simulink model "main_savepoint"  (R2021a)
settings: Solver=VariableStepAuto  StartTime=0.0  StopTime=60  RelTol=1e-3
undefined symbols (not defined in the file or in its folder): Earth, WGS84
libraries: pid_lib x6, dspvision x5, dspindex x2, aerolibfltsims x1, aerolibtransform2 x1, dspsnks4 x1, simulink x1
settings Model: Creator=ZumoArthicha  LastModifiedBy=ZumoArthicha

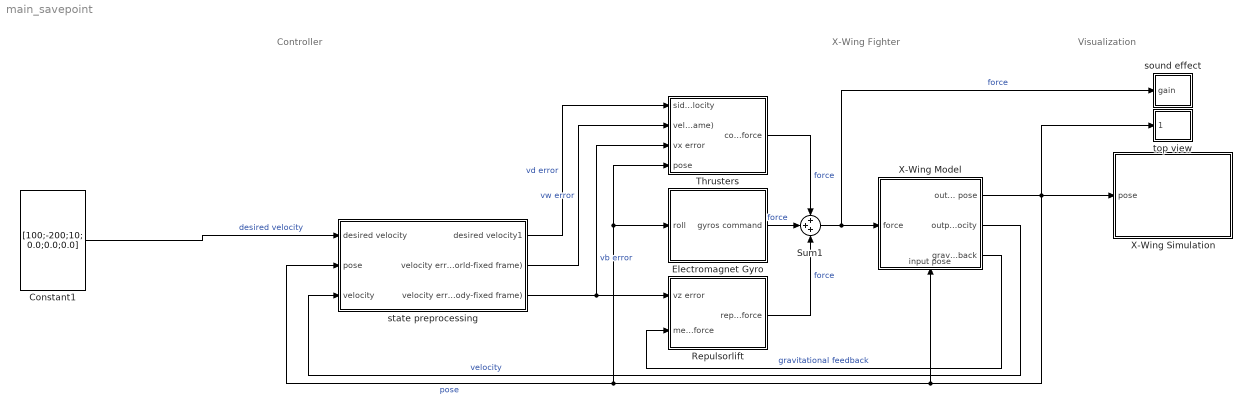
== system main_savepoint ==
  note: Controller
  note: Visualization
  note: X-Wing Fighter
  Constant1 : Constant  Value=[100;-200;10; 0.0;0.0;0.0]  VectorParams1D=off
  Electromagnet Gyro : Subsystem
      mask Display: image(imread("pictures/electromagneticgyro.PNG"))
  Repulsorlift : Subsystem
      mask Display: image(imread("pictures/repulserlift.PNG"))
  Sum1 : Sum  Inputs=+++
  Thrusters : Subsystem
      mask Display: image(imread("pictures/thrusters.PNG"))
  X-Wing Model : Subsystem
      settings: PortSchema="{\"entries\":[{\"content\":{\"sides\":[{\"content\":{\"connectorIds\":[\"In1\"]},\"type\":\"ConnectorPlacement.EquallySpacedRectSide\",\"uuid\":\"9b8fdf7d-c3f6-4599-b802-210579db8a0c\"},{\"content\":{\"connectorIds\":[\"Out1\",\"Out2\",\"Out3\"],\"side\":\"RIGHT\"},\"type\":\"ConnectorPlacement.EquallySpacedRectSide\",\"uuid\":\"64fce1f1-7921-46e2-bebf-614926f0f3ad\"},{\"content\":{\"connectorIds\":[],\"side\":\"TOP\"},\"type\":\"ConnectorPlacement.EquallySpacedRectSide\",\"uuid\":\"e545f28f-71e6-4ea6-95f8-1eb7e380d19b\"},{\"content\":{\"connectorIds\":[\"In2\"],\"side\":\"BOTTOM\"},\"type\":\"ConnectorPlacement.EquallySpacedRectSide\",\"uuid\":\"bfd9a8ec-cd4d-4e0d-ab0a-253386349908\"}]},\"type\":\"ConnectorPlacement.EquallySpacedConnector\",\"uuid\":\"b40ebf44-1443-4f81-b67e-9daee8e56b53\"}],\"packageUris\":[\"http://schema.mathworks.com/mf0/Connector/R2020b\"],\"version\":\"1.0\"}"
      mask Display: image(imread("pictures/simplified_model.png"))
  X-Wing Simulation : Subsystem
      mask Display: image(imread("pictures/simulation.PNG"))
  sound effect : Subsystem
      mask Display: image(imread("pictures/audio.PNG"))
  state preprocessing : Subsystem
  top view : Subsystem
      mask Display: image(imread("pictures/xy_graph.png"))
  wires:
  X-Wing Model/1(output pose) -> state preprocessing/2(pose), Electromagnet Gyro/1(roll), Thrusters/4(pose), X-Wing Model/2(input pose), X-Wing Simulation/1(pose), top view/1(" ")  "pose"
  X-Wing Model/3(gravitational force feedback) -> Repulsorlift/2(measured gravity force)  "gravitational feedback"
  Thrusters/1(combined thrusters force) -> Sum1/1  "force"
  Sum1/1 -> sound effect/1(gain), X-Wing Model/1(force)  "force"
  Electromagnet Gyro/1(gyros command) -> Sum1/2  "force"
  Repulsorlift/1(repulsorlift force) -> Sum1/3  "force"
  state preprocessing/3(velocity error (body-fixed frame)) -> Thrusters/3(vx error), Repulsorlift/1(vz error)  "vb error"
  X-Wing Model/2(output veloocity) -> state preprocessing/3(velocity)  "velocity"
  Constant1/1 -> state preprocessing/1(desired velocity)  "desired velocity"
  state preprocessing/1(desired velocity1) -> Thrusters/1(sideway velocity)  "vd error"
  state preprocessing/2(velocity error (world-fixed frame)) -> Thrusters/2(velocity error (world-fixed frame))  "vw error"

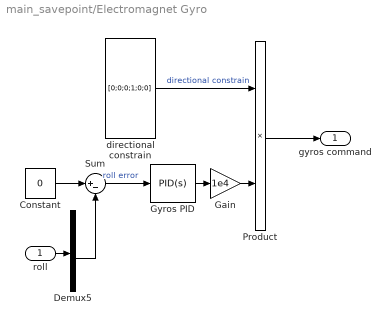
== system main_savepoint/Electromagnet Gyro ==
  roll : Inport
  Constant : Constant  Value=0
  Demux5 : Demux  Outputs=6
  Gain : Gain  Gain=1e4
  Gyros PID : pid_lib/PID Controller  Controller=PID  Form=Parallel  TimeDomain=Continuous-time  UseExternalTs=off  SampleTime=-1  IntegratorMethod=Forward Euler  FilterMethod=Forward Euler  ControllerParametersSource=internal  P=0.1  I=0  D=1  UseFilter=on  N=100  TunerSelectOption=Transfer Function Based (PID Tuner App)  InitialConditionSource=internal  InitialConditionForIntegrator=0  InitialConditionForFilter=0  DifferentiatorICPrevScaledInput=0  ExternalReset=none  TrackingMode=off  Kt=1  LimitOutput=off  SatLimitsSource=internal  UpperSaturationLimit=inf  LowerSaturationLimit=-inf  LinearizeAsGain=on  AntiWindupMode=none  Kb=1  POutMin=[]  POutMax=[]  IOutMin=[]  IOutMax=[]  DOutMin=[]  DOutMax=[]  NOutMin=[]  NOutMax=[]  SumOutMin=[]  SumOutMax=[]  SaturationOutMin=[]  SaturationOutMax=[]  PParamMin=[]  PParamMax=[]  IParamMin=[]  IParamMax=[]  DParamMin=[]  DParamMax=[]  NParamMin=[]  NParamMax=[]  KbParamMin=[]  KbParamMax=[]  KtParamMin=[]  KtParamMax=[]  KbOutMin=[]  KbOutMax=[]  KtOutMin=[]  KtOutMax=[]  IntegratorOutMin=[]  IntegratorOutMax=[]  FilterOutMin=[]  FilterOutMax=[]  SumI1OutMin=[]  SumI1OutMax=[]  SumI2OutMin=[]  SumI2OutMax=[]  SumI3OutMin=[]  SumI3OutMax=[]  SumI4OutMin=[]  SumI4OutMax=[]  SumDOutMin=[]  SumDOutMax=[]  DifferentiatorOutMin=[]  DifferentiatorOutMax=[]  FilterDiffOutCoefMin=[]  FilterDiffOutCoefMax=[]  ReciprocalOutMin=[]  ReciprocalOutMax=[]  SumDenOutMin=[]  SumDenOutMax=[]  SumNumOutMin=[]  SumNumOutMax=[]  DivideOutMin=[]  DivideOutMax=[]  UdiffTsProdOutMin=[]  UdiffTsProdOutMax=[]  NTsProdOutMin=[]  NTsProdOutMax=[]  UintegralTsProdOutMin=[]  UintegralTsProdOutMax=[]  UngainTsProdOutMin=[]  UngainTsProdOutMax=[]  IntegratorContinuousStateAttributes=''  IntegratorStateMustResolveToSignalObject=off  IntegratorRTWStateStorageClass=Auto  FilterContinuousStateAttributes=''  FilterStateMustResolveToSignalObject=off  FilterRTWStateStorageClass=Auto  ParallelPVariant=InternalParameters  IdealPVariant=Disabled  IVariant=InternalParameters  DVariant=InternalParameters  IntegratorVariant=Continuous  SatVariant=Disabled  AWVariant=Passthrough  PCopyVariant=Disabled  TRVariant=Disabled  FdbkBlocksVariant=Forward  IdealPFdbkVariant=Disabled  SatFdbkVariant=Disabled  DerivativeFilterVariant=ContFilter  NVariant=InternalParameters  NCopyVariant=Disabled  FilterICVariant=InternalICsFilter  IntegratorICVariant=InternalICs  ExternalResetVariant=Disabled  TRSumVariant=Passthrough  SumFdbkVariant=Disabled  SumVariant=Sum_PID  TsampFilterVariant=InternalTs  TsampNgainVariant=Passthrough  TsampIntegralVariant=Passthrough  ExternalSaturationOutDataTypeStr=Inherit: Same as second input
  Product : Product
  Sum : Sum  Inputs=|+-
  directional constrain : Constant  Value=[0;0;0;1;0;0]  VectorParams1D=off
  gyros command : Outport  PortDimensions=6
  wires:
  directional constrain/1 -> Product/1  "directional constrain"
  Gyros PID/1 -> Gain/1
  Product/1 -> gyros command/1
  Gain/1 -> Product/2
  Sum/1 -> Gyros PID/1  "roll error"
  Constant/1 -> Sum/1
  roll/1 -> Demux5/1
  Demux5/4 -> Sum/2

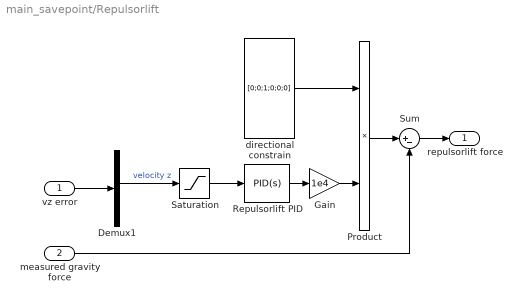
== system main_savepoint/Repulsorlift ==
  vz error : Inport
  measured gravity force : Inport  Port=2
  Demux1 : Demux  Outputs=6
  Gain : Gain  Gain=1e4
  Product : Product
  Repulsorlift PID : pid_lib/PID Controller  Controller=PID  Form=Parallel  TimeDomain=Continuous-time  UseExternalTs=off  SampleTime=-1  IntegratorMethod=Forward Euler  FilterMethod=Forward Euler  ControllerParametersSource=internal  P=0.05  I=0  D=1  UseFilter=on  N=100  TunerSelectOption=Transfer Function Based (PID Tuner App)  InitialConditionSource=internal  InitialConditionForIntegrator=0  InitialConditionForFilter=0  DifferentiatorICPrevScaledInput=0  ExternalReset=none  TrackingMode=off  Kt=1  LimitOutput=off  SatLimitsSource=internal  UpperSaturationLimit=inf  LowerSaturationLimit=-inf  LinearizeAsGain=on  AntiWindupMode=none  Kb=1  POutMin=[]  POutMax=[]  IOutMin=[]  IOutMax=[]  DOutMin=[]  DOutMax=[]  NOutMin=[]  NOutMax=[]  SumOutMin=[]  SumOutMax=[]  SaturationOutMin=[]  SaturationOutMax=[]  PParamMin=[]  PParamMax=[]  IParamMin=[]  IParamMax=[]  DParamMin=[]  DParamMax=[]  NParamMin=[]  NParamMax=[]  KbParamMin=[]  KbParamMax=[]  KtParamMin=[]  KtParamMax=[]  KbOutMin=[]  KbOutMax=[]  KtOutMin=[]  KtOutMax=[]  IntegratorOutMin=[]  IntegratorOutMax=[]  FilterOutMin=[]  FilterOutMax=[]  SumI1OutMin=[]  SumI1OutMax=[]  SumI2OutMin=[]  SumI2OutMax=[]  SumI3OutMin=[]  SumI3OutMax=[]  SumI4OutMin=[]  SumI4OutMax=[]  SumDOutMin=[]  SumDOutMax=[]  DifferentiatorOutMin=[]  DifferentiatorOutMax=[]  FilterDiffOutCoefMin=[]  FilterDiffOutCoefMax=[]  ReciprocalOutMin=[]  ReciprocalOutMax=[]  SumDenOutMin=[]  SumDenOutMax=[]  SumNumOutMin=[]  SumNumOutMax=[]  DivideOutMin=[]  DivideOutMax=[]  UdiffTsProdOutMin=[]  UdiffTsProdOutMax=[]  NTsProdOutMin=[]  NTsProdOutMax=[]  UintegralTsProdOutMin=[]  UintegralTsProdOutMax=[]  UngainTsProdOutMin=[]  UngainTsProdOutMax=[]  IntegratorContinuousStateAttributes=''  IntegratorStateMustResolveToSignalObject=off  IntegratorRTWStateStorageClass=Auto  FilterContinuousStateAttributes=''  FilterStateMustResolveToSignalObject=off  FilterRTWStateStorageClass=Auto  ParallelPVariant=InternalParameters  IdealPVariant=Disabled  IVariant=InternalParameters  DVariant=InternalParameters  IntegratorVariant=Continuous  SatVariant=Disabled  AWVariant=Passthrough  PCopyVariant=Disabled  TRVariant=Disabled  FdbkBlocksVariant=Forward  IdealPFdbkVariant=Disabled  SatFdbkVariant=Disabled  DerivativeFilterVariant=ContFilter  NVariant=InternalParameters  NCopyVariant=Disabled  FilterICVariant=InternalICsFilter  IntegratorICVariant=InternalICs  ExternalResetVariant=Disabled  TRSumVariant=Passthrough  SumFdbkVariant=Disabled  SumVariant=Sum_PID  TsampFilterVariant=InternalTs  TsampNgainVariant=Passthrough  TsampIntegralVariant=Passthrough  ExternalSaturationOutDataTypeStr=Inherit: Same as second input
  Saturation : Saturate  UpperLimit=1  LowerLimit=-1
  Sum : Sum  Inputs=|+-
  directional constrain : Constant  Value=[0;0;1;0;0;0]  VectorParams1D=off
  repulsorlift force : Outport  PortDimensions=6
  wires:
  directional constrain/1 -> Product/1
  Repulsorlift PID/1 -> Gain/1
  Product/1 -> Sum/1
  Sum/1 -> repulsorlift force/1
  Gain/1 -> Product/2
  measured gravity force/1 -> Sum/2
  Saturation/1 -> Repulsorlift PID/1
  vz error/1 -> Demux1/1
  Demux1/3 -> Saturation/1  "velocity z"

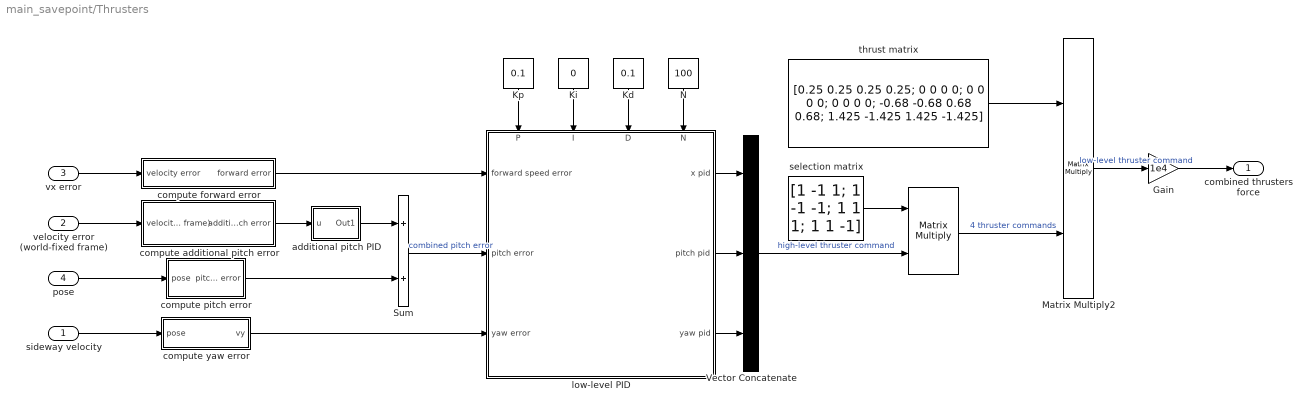
== system main_savepoint/Thrusters ==
  sideway velocity : Inport
  velocity error (world-fixed frame) : Inport  Port=2
  vx error : Inport  Port=3
  pose : Inport  Port=4
  "  " : Product  Multiplication=Matrix(*)
  Gain : Gain  Gain=1e4
  Kd : Constant  Value=0.1
  Ki : Constant  Value=0
  Kp : Constant  Value=0.1
  Matrix Multiply2 : Product  Multiplication=Matrix(*)
  N : Constant  Value=100
  Sum : Sum
  Vector Concatenate : Concatenate  NumInputs=3
  additional pitch PID : Subsystem
  compute additional pitch error : Subsystem
  compute forward error : Subsystem
  compute pitch error : Subsystem
  compute yaw error : Subsystem
  low-level PID : Subsystem
      settings: PortSchema="{\"entries\":[{\"content\":{\"sides\":[{\"content\":{\"connectorIds\":[\"In1\",\"In2\",\"In3\"]},\"type\":\"ConnectorPlacement.EquallySpacedRectSide\",\"uuid\":\"f6ea6f6d-4efd-425d-8a85-ce3b9bde565c\"},{\"content\":{\"connectorIds\":[\"Out1\",\"Out2\",\"Out3\"],\"side\":\"RIGHT\"},\"type\":\"ConnectorPlacement.EquallySpacedRectSide\",\"uuid\":\"bea2efba-fcca-41fe-8e46-9fa204d644b4\"},{\"content\":{\"connectorIds\":[\"In4\",\"In5\",\"In6\",\"In7\"],\"side\":\"TOP\"},\"type\":\"ConnectorPlacement.EquallySpacedRectSide\",\"uuid\":\"c7db24d1-2300-4d89-a06d-38d8ccf635f0\"}]},\"type\":\"ConnectorPlacement.EquallySpacedConnector\",\"uuid\":\"54c313d2-af5a-49ea-a2f4-4d36f80b668a\"}],\"packageUris\":[\"http://schema.mathworks.com/mf0/Connector/R2020b\"],\"version\":\"1.0\"}"
  selection matrix : Constant  Value=[1 -1 1; 1 -1 -1; 1 1 1; 1 1 -1]  VectorParams1D=off
  thrust matrix : Constant  Value=[0.25 0.25 0.25 0.25; 0 0 0 0; 0 0 0 0; 0 0 0 0; -0.68 -0.68 0.68 0.68; 1.425 -1.425 1.425 -1.425]  VectorParams1D=off
  combined thrusters force : Outport  PortDimensions=6
  wires:
  Kp/1 -> low-level PID/4(P)
  selection matrix/1 -> "  "/1
  Gain/1 -> combined thrusters force/1
  thrust matrix/1 -> Matrix Multiply2/1
  Vector Concatenate/1 -> "  "/2  "high-level thruster command"
  "  "/1 -> Matrix Multiply2/2  "4 thruster commands"
  Matrix Multiply2/1 -> Gain/1  "low-level thruster command"
  pose/1 -> compute pitch error/1(pose)
  compute pitch error/1(pitch error) -> Sum/2
  vx error/1 -> compute forward error/1(velocity error)
  velocity error (world-fixed frame)/1 -> compute additional pitch error/1(velocity error (world-fixed frame))
  sideway velocity/1 -> compute yaw error/1(pose)
  compute additional pitch error/1(addition pitch error) -> additional pitch PID/1(u)
  additional pitch PID/1(Out1) -> Sum/1
  Ki/1 -> low-level PID/5(I)
  Kd/1 -> low-level PID/6(D)
  N/1 -> low-level PID/7(N)
  compute forward error/1(forward error) -> low-level PID/1(forward speed error)
  Sum/1 -> low-level PID/2(pitch error)  "combined pitch error"
  compute yaw error/1(vy) -> low-level PID/3(yaw error)
  low-level PID/1(x pid) -> Vector Concatenate/1
  low-level PID/2(pitch pid) -> Vector Concatenate/2
  low-level PID/3(yaw pid) -> Vector Concatenate/3

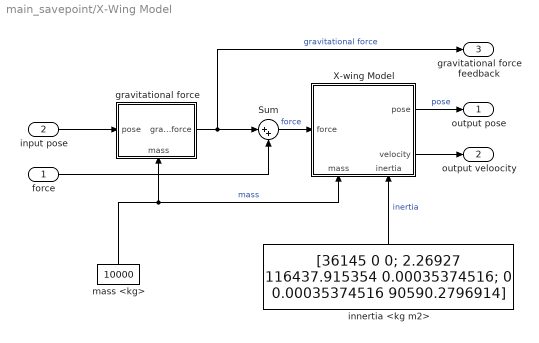
== system main_savepoint/X-Wing Model ==
  force : Inport
  input pose : Inport  Port=2
  Sum : Sum  Inputs=|++
  X-wing Model : Subsystem
      settings: PortSchema="{\"entries\":[{\"content\":{\"sides\":[{\"content\":{\"connectorIds\":[\"In1\"]},\"type\":\"ConnectorPlacement.EquallySpacedRectSide\",\"uuid\":\"7004d7e2-eb30-41ed-9d5e-f00159415fc4\"},{\"content\":{\"connectorIds\":[\"Out1\",\"Out2\"],\"side\":\"RIGHT\"},\"type\":\"ConnectorPlacement.EquallySpacedRectSide\",\"uuid\":\"4cf7ba01-0c86-439c-9faf-473746ab50fc\"},{\"content\":{\"connectorIds\":[],\"side\":\"TOP\"},\"type\":\"ConnectorPlacement.EquallySpacedRectSide\",\"uuid\":\"4a15a873-16d7-4740-9282-1fecb26c48e4\"},{\"content\":{\"connectorIds\":[\"In2\",\"In3\"],\"side\":\"BOTTOM\"},\"type\":\"ConnectorPlacement.EquallySpacedRectSide\",\"uuid\":\"87e73f3e-eb46-42cc-8158-d40318a5aa75\"}]},\"type\":\"ConnectorPlacement.EquallySpacedConnector\",\"uuid\":\"64dad74e-3dd4-4677-9bab-84aaaaaa8f26\"}],\"packageUris\":[\"http://schema.mathworks.com/mf0/Connector/R2020b\"],\"version\":\"1.0\"}"
      mask Display: image(imread("pictures/simplified_model.png"))
  gravitational force : Subsystem
      settings: PortSchema="{\"entries\":[{\"content\":{\"sides\":[{\"content\":{\"connectorIds\":[\"In1\"]},\"type\":\"ConnectorPlacement.EquallySpacedRectSide\",\"uuid\":\"d93db66b-fcc6-4c17-9134-40d9beba2643\"},{\"content\":{\"connectorIds\":[\"Out1\"],\"side\":\"RIGHT\"},\"type\":\"ConnectorPlacement.EquallySpacedRectSide\",\"uuid\":\"70571ecc-e0da-42b3-8b7b-d4ce677f32d8\"},{\"content\":{\"connectorIds\":[],\"side\":\"TOP\"},\"type\":\"ConnectorPlacement.EquallySpacedRectSide\",\"uuid\":\"56b2d7be-0ac4-47dc-afb8-3ce057fd0ced\"},{\"content\":{\"connectorIds\":[\"In2\"],\"side\":\"BOTTOM\"},\"type\":\"ConnectorPlacement.EquallySpacedRectSide\",\"uuid\":\"175b75d5-a12f-4632-9256-2a0db7457e72\"}]},\"type\":\"ConnectorPlacement.EquallySpacedConnector\",\"uuid\":\"6f54763d-dba9-4fd6-aa24-fb7b6af2d4a1\"}],\"packageUris\":[\"http://schema.mathworks.com/mf0/Connector/R2020b\"],\"version\":\"1.0\"}"
      mask Display: image(imread("pictures/gravitational_force.PNG"))
  innertia <kg m2> : Constant  Value=[36145 0 0; 2.26927 116437.915354 0.00035374516; 0 0.00035374516 90590.2796914]  VectorParams1D=off
  mass <kg> : Constant  Value=10000
  output pose : Outport
  output veloocity : Outport  Port=2
  gravitational force feedback : Outport  Port=3
  wires:
  mass <kg>/1 -> gravitational force/2(mass), X-wing Model/2(mass)  "mass"
  innertia <kg m2>/1 -> X-wing Model/3(inertia)  "inertia"
  X-wing Model/1(pose) -> output pose/1  "pose"
  input pose/1 -> gravitational force/1(pose)
  Sum/1 -> X-wing Model/1(force)  "force"
  force/1 -> Sum/2
  gravitational force/1(gravitational force) -> gravitational force feedback/1, Sum/1  "gravitational force"
  X-wing Model/2(velocity) -> output veloocity/1

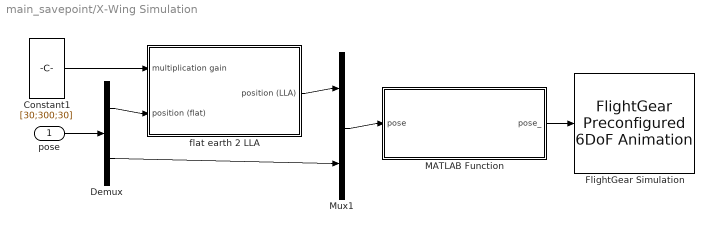
== system main_savepoint/X-Wing Simulation ==
  pose : Inport
  Constant1 : Constant  Value=[30;300;30]  VectorParams1D=off
  Demux : Demux  Outputs=2
  FlightGear Simulation : aerolibfltsims/FlightGear Preconfigured 6DoF Animation  xFlightGearVersion=v2019.1  DestinationIpAddress=127.0.0.1  DestinationPort=5502  SampleTime=1/30  packetVersion=24  mask(FlightGearQuick6DoFAnimation){}
      mask Display:
      | % This is a new mask on top of the base mask.
      | % Use "View base mask" link below to see the base mask.
      | image(imread("pictures/simulation.PNG"))
  MATLAB Function : MATLAB Function  TreatAsAtomicUnit=on
  Mux1 : Mux  Inputs=2
  flat earth 2 LLA : Subsystem
  wires:
  MATLAB Function/1(pose_) -> FlightGear Simulation/1
  pose/1 -> Demux/1
  Demux/2 -> Mux1/2
  Mux1/1 -> MATLAB Function/1(pose)
  Constant1/1 -> flat earth 2 LLA/1(multiplication gain)
  Demux/1 -> flat earth 2 LLA/2(position (flat))
  flat earth 2 LLA/1(position (LLA)) -> Mux1/1

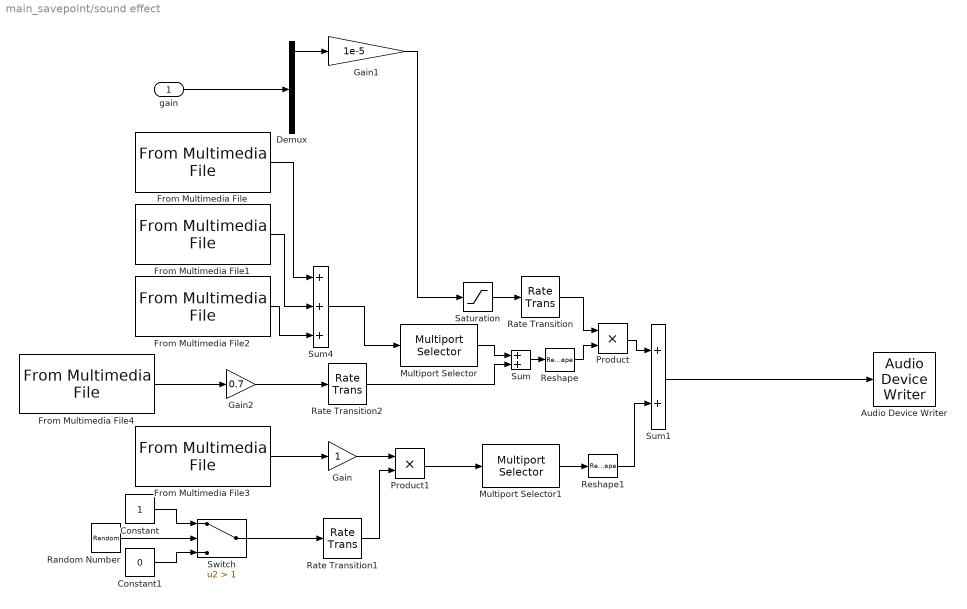
== system main_savepoint/sound effect ==
  gain : Inport
  Audio Device Writer : dspsnks4/Audio Device Writer  Driver=DirectSound  Device=Default  InheritSampleRate=on  SampleRate=44100  BitDepth=16-bit integer  BufferSize=4096  NumBuffers=10  DefaultOutputChannelMapping=on  OutputChannelMapping=1:2  OutputNumUnderrunSamples=off  DriverIdx=1  DeviceWarnFlag=''
  Constant : Constant
  Constant1 : Constant  Value=0
  Demux : Demux  Outputs=6
  From Multimedia File : dspvision/From Multimedia File  inputFilename=D:\SDU\courses\F22_GuidanceNavigationAndControl\project\workspace\sound\XWing-Fly1.wav  readRange=[1 Inf]  loop=on  numPlays=inf  outputStreams=Audio only  videoDataType=single  audioDataType=double  inheritSampleTime=on  userDefinedSampleTime=1/30  noAudioOutput=off  isIntensityVideo=off  fourcc=RGB  colorVideoFormat=One multidimensional signal  outputEOF=off  dataOrg=Column-major  audioFrameSize=1024  computeAudioFrameSize=off  outSamplingMode=Sample based
  From Multimedia File1 : dspvision/From Multimedia File  inputFilename=D:\SDU\courses\F22_GuidanceNavigationAndControl\project\workspace\sound\XWing-Fly2.wav  readRange=[1 Inf]  loop=on  numPlays=inf  outputStreams=Audio only  videoDataType=single  audioDataType=double  inheritSampleTime=on  userDefinedSampleTime=1/30  noAudioOutput=off  isIntensityVideo=off  fourcc=RGB  colorVideoFormat=One multidimensional signal  outputEOF=off  dataOrg=Column-major  audioFrameSize=1024  computeAudioFrameSize=off  outSamplingMode=Sample based
  From Multimedia File2 : dspvision/From Multimedia File  inputFilename=D:\SDU\courses\F22_GuidanceNavigationAndControl\project\workspace\sound\XWing-Fly3.wav  readRange=[1 Inf]  loop=on  numPlays=inf  outputStreams=Audio only  videoDataType=single  audioDataType=double  inheritSampleTime=on  userDefinedSampleTime=1/30  noAudioOutput=off  isIntensityVideo=off  fourcc=RGB  colorVideoFormat=One multidimensional signal  outputEOF=off  dataOrg=Column-major  audioFrameSize=1024  computeAudioFrameSize=off  outSamplingMode=Sample based
  From Multimedia File3 : dspvision/From Multimedia File  inputFilename=D:\SDU\courses\F22_GuidanceNavigationAndControl\project\workspace\sound\XWing-Laser.wav  readRange=[1 Inf]  loop=on  numPlays=inf  outputStreams=Audio only  videoDataType=single  audioDataType=double  inheritSampleTime=on  userDefinedSampleTime=1/30  noAudioOutput=off  isIntensityVideo=off  fourcc=RGB  colorVideoFormat=One multidimensional signal  outputEOF=off  dataOrg=Column-major  audioFrameSize=1024  computeAudioFrameSize=off  outSamplingMode=Sample based
  From Multimedia File4 : dspvision/From Multimedia File  inputFilename=D:\SDU\courses\F22_GuidanceNavigationAndControl\project\workspace\sound\R2D2.mp3  readRange=[1 Inf]  loop=on  numPlays=inf  outputStreams=Audio only  videoDataType=single  audioDataType=double  inheritSampleTime=on  userDefinedSampleTime=1/30  noAudioOutput=off  isIntensityVideo=off  fourcc=RGB  colorVideoFormat=One multidimensional signal  outputEOF=off  dataOrg=Column-major  audioFrameSize=1024  computeAudioFrameSize=off  outSamplingMode=Sample based
  Gain : Gain
  Gain1 : Gain  Gain=1e-5
  Gain2 : Gain  Gain=0.7
  Multiport Selector : dspindex/Multiport Selector  rowsOrCols=Columns  idxCellArray=2  idxErrMode=Clip Index
  Multiport Selector1 : dspindex/Multiport Selector  rowsOrCols=Columns  idxCellArray=2  idxErrMode=Clip Index
  Product : Product
  Product1 : Product
  Random Number : RandomNumber  SampleTime=0.4643990929705216
  Rate Transition : RateTransition
  Rate Transition1 : RateTransition
  Rate Transition2 : RateTransition
  Reshape : Reshape
  Reshape1 : Reshape
  Saturation : Saturate  UpperLimit=1  LowerLimit=0.5
  Sum : Sum
  Sum1 : Sum
  Sum4 : Sum  Inputs=+++
  Switch : Switch  Criteria=u2 > Threshold  Threshold=1
  wires:
  From Multimedia File3/1 -> Gain/1
  From Multimedia File/1 -> Sum4/1
  From Multimedia File2/1 -> Sum4/3
  From Multimedia File1/1 -> Sum4/2
  Product/1 -> Sum1/1
  Sum1/1 -> Audio Device Writer/1
  Sum4/1 -> Multiport Selector/1
  Multiport Selector1/1 -> Reshape1/1
  Demux/1 -> Gain1/1
  gain/1 -> Demux/1
  Gain1/1 -> Saturation/1
  Rate Transition/1 -> Product/1
  Reshape1/1 -> Sum1/2
  Saturation/1 -> Rate Transition/1
  Gain/1 -> Product1/1
  Product1/1 -> Multiport Selector1/1
  Rate Transition1/1 -> Product1/2
  Random Number/1 -> Switch/2
  Constant/1 -> Switch/1
  Constant1/1 -> Switch/3
  Switch/1 -> Rate Transition1/1
  From Multimedia File4/1 -> Gain2/1
  Reshape/1 -> Product/2
  Sum/1 -> Reshape/1
  Multiport Selector/1 -> Sum/1
  Rate Transition2/1 -> Sum/2
  Gain2/1 -> Rate Transition2/1

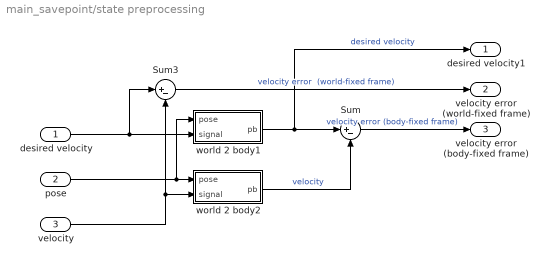
== system main_savepoint/state preprocessing ==
  desired velocity : Inport
  pose : Inport  Port=2
  velocity : Inport  Port=3
  Sum : Sum  Inputs=|+-
  Sum3 : Sum  Inputs=|+-
  world 2 body1 : MATLAB Function  TreatAsAtomicUnit=on
  world 2 body2 : MATLAB Function  TreatAsAtomicUnit=on
  desired velocity1 : Outport
  velocity error (world-fixed frame) : Outport  Port=2
  velocity error (body-fixed frame) : Outport  Port=3
  wires:
  velocity/1 -> world 2 body2/2(signal), Sum3/2
  world 2 body1/1(pb) -> desired velocity1/1, Sum/1  "desired velocity"
  desired velocity/1 -> world 2 body1/2(signal), Sum3/1
  Sum/1 -> velocity error (body-fixed frame)/1  "velocity error (body-fixed frame)"
  pose/1 -> world 2 body1/1(pose), world 2 body2/1(pose)
  world 2 body2/1(pb) -> Sum/2  "velocity"
  Sum3/1 -> velocity error (world-fixed frame)/1  "velocity error  (world-fixed frame)"

== system main_savepoint/top view ==
  " " : Inport
  Demux3 : Demux  Outputs=6
  XY Graph : simulink/Sinks/XY Graph  xmin=-1  xmax=1  ymin=-1  ymax=1  st=-1
  scaling gain : Gain  Gain=1e-4
  wires:
  Demux3/1 -> XY Graph/1  "x"
  Demux3/2 -> XY Graph/2  "y"
  scaling gain/1 -> Demux3/1
  " "/1 -> scaling gain/1

== system main_savepoint/Thrusters/additional pitch PID ==
  u : Inport
  Gain1 : Gain  Gain=-1
  pitch PID1 : pid_lib/PID Controller  Controller=PID  Form=Parallel  TimeDomain=Continuous-time  UseExternalTs=off  SampleTime=-1  IntegratorMethod=Forward Euler  FilterMethod=Forward Euler  ControllerParametersSource=internal  P=1e-2  I=0  D=0.01  UseFilter=on  N=100  TunerSelectOption=Transfer Function Based (PID Tuner App)  InitialConditionSource=internal  InitialConditionForIntegrator=0  InitialConditionForFilter=0  DifferentiatorICPrevScaledInput=0  ExternalReset=none  TrackingMode=off  Kt=1  LimitOutput=off  SatLimitsSource=internal  UpperSaturationLimit=inf  LowerSaturationLimit=-inf  LinearizeAsGain=on  AntiWindupMode=none  Kb=1  POutMin=[]  POutMax=[]  IOutMin=[]  IOutMax=[]  DOutMin=[]  DOutMax=[]  NOutMin=[]  NOutMax=[]  SumOutDataTypeStr=double  SumOutMin=[]  SumOutMax=[]  SaturationOutMin=[]  SaturationOutMax=[]  PParamMin=[]  PParamMax=[]  IParamMin=[]  IParamMax=[]  DParamMin=[]  DParamMax=[]  NParamMin=[]  NParamMax=[]  KbParamMin=[]  KbParamMax=[]  KtParamMin=[]  KtParamMax=[]  KbOutMin=[]  KbOutMax=[]  KtOutMin=[]  KtOutMax=[]  IntegratorOutMin=[]  IntegratorOutMax=[]  FilterOutMin=[]  FilterOutMax=[]  SumI1OutMin=[]  SumI1OutMax=[]  SumI2OutMin=[]  SumI2OutMax=[]  SumI3OutMin=[]  SumI3OutMax=[]  SumI4OutMin=[]  SumI4OutMax=[]  SumDOutMin=[]  SumDOutMax=[]  DifferentiatorOutMin=[]  DifferentiatorOutMax=[]  FilterDiffOutCoefMin=[]  FilterDiffOutCoefMax=[]  ReciprocalOutMin=[]  ReciprocalOutMax=[]  SumDenOutMin=[]  SumDenOutMax=[]  SumNumOutMin=[]  SumNumOutMax=[]  DivideOutMin=[]  DivideOutMax=[]  UdiffTsProdOutMin=[]  UdiffTsProdOutMax=[]  NTsProdOutMin=[]  NTsProdOutMax=[]  UintegralTsProdOutMin=[]  UintegralTsProdOutMax=[]  UngainTsProdOutMin=[]  UngainTsProdOutMax=[]  IntegratorContinuousStateAttributes=''  IntegratorStateMustResolveToSignalObject=off  IntegratorRTWStateStorageClass=Auto  FilterContinuousStateAttributes=''  FilterStateMustResolveToSignalObject=off  FilterRTWStateStorageClass=Auto  ParallelPVariant=InternalParameters  IdealPVariant=Disabled  IVariant=InternalParameters  DVariant=InternalParameters  IntegratorVariant=Continuous  SatVariant=Disabled  AWVariant=Passthrough  PCopyVariant=Disabled  TRVariant=Disabled  FdbkBlocksVariant=Forward  IdealPFdbkVariant=Disabled  SatFdbkVariant=Disabled  DerivativeFilterVariant=ContFilter  NVariant=InternalParameters  NCopyVariant=Disabled  FilterICVariant=InternalICsFilter  IntegratorICVariant=InternalICs  ExternalResetVariant=Disabled  TRSumVariant=Passthrough  SumFdbkVariant=Disabled  SumVariant=Sum_PID  TsampFilterVariant=InternalTs  TsampNgainVariant=Passthrough  TsampIntegralVariant=Passthrough  ExternalSaturationOutDataTypeStr=Inherit: Same as second input
  Out1 : Outport  PortDimensions=1
  wires:
  Gain1/1 -> Out1/1
  pitch PID1/1 -> Gain1/1
  u/1 -> pitch PID1/1

== system main_savepoint/Thrusters/compute additional pitch error ==
  velocity error (world-fixed frame) : Inport
  Abs : Abs
  Constant : Constant  Value=0
  Demux4 : Demux  Outputs=6
  Saturation : Saturate  UpperLimit=10  LowerLimit=-10
  Switch : Switch  Criteria=u2 > Threshold  Threshold=5
  addition pitch error : Outport  PortDimensions=1
  wires:
  Demux4/3 -> Abs/1, Switch/1
  Abs/1 -> Switch/2
  Constant/1 -> Switch/3
  Switch/1 -> Saturation/1
  Saturation/1 -> addition pitch error/1
  velocity error (world-fixed frame)/1 -> Demux4/1

== system main_savepoint/Thrusters/compute forward error ==
  velocity error : Inport
  Demux1 : Demux  Outputs=6
  forward error : Outport
  wires:
  Demux1/1 -> forward error/1
  velocity error/1 -> Demux1/1

== system main_savepoint/Thrusters/compute pitch error ==
  pose : Inport
  Constant2 : Constant  Value=0
  Demux5 : Demux  Outputs=6
  Sum1 : Sum  Inputs=|+-
  pitch error : Outport
  wires:
  Demux5/5 -> Sum1/2  "pitch"
  pose/1 -> Demux5/1
  Constant2/1 -> Sum1/1
  Sum1/1 -> pitch error/1  "pitch error"

== system main_savepoint/Thrusters/compute yaw error ==
  pose : Inport
  Demux2 : Demux  Outputs=6
  vy : Outport
  wires:
  pose/1 -> Demux2/1
  Demux2/2 -> vy/1  "vy"

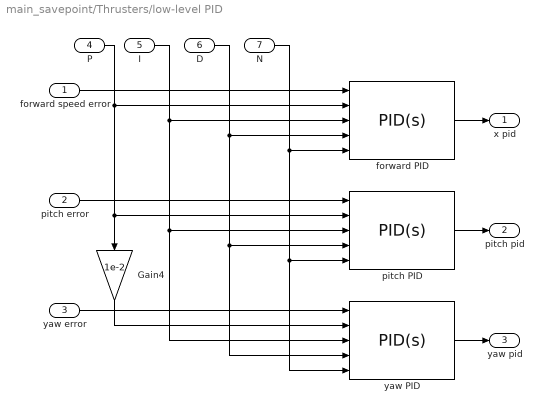
== system main_savepoint/Thrusters/low-level PID ==
  forward speed error : Inport
  pitch error : Inport  Port=2
  yaw error : Inport  Port=3
  P : Inport  Port=4
  I : Inport  Port=5
  D : Inport  Port=6
  N : Inport  Port=7
  Gain4 : Gain  Gain=1e-2
  forward PID : pid_lib/PID Controller  Controller=PID  Form=Parallel  TimeDomain=Continuous-time  UseExternalTs=off  SampleTime=-1  IntegratorMethod=Forward Euler  FilterMethod=Forward Euler  ControllerParametersSource=external  P=0.01  I=0  D=1  UseFilter=on  N=100  TunerSelectOption=Transfer Function Based (PID Tuner App)  InitialConditionSource=internal  InitialConditionForIntegrator=0  InitialConditionForFilter=0  DifferentiatorICPrevScaledInput=0  ExternalReset=none  TrackingMode=off  Kt=1  LimitOutput=off  SatLimitsSource=internal  UpperSaturationLimit=inf  LowerSaturationLimit=-inf  LinearizeAsGain=on  AntiWindupMode=none  Kb=1  POutMin=[]  POutMax=[]  IOutMin=[]  IOutMax=[]  DOutMin=[]  DOutMax=[]  NOutMin=[]  NOutMax=[]  SumOutMin=[]  SumOutMax=[]  SaturationOutMin=[]  SaturationOutMax=[]  PParamMin=[]  PParamMax=[]  IParamMin=[]  IParamMax=[]  DParamMin=[]  DParamMax=[]  NParamMin=[]  NParamMax=[]  KbParamMin=[]  KbParamMax=[]  KtParamMin=[]  KtParamMax=[]  KbOutMin=[]  KbOutMax=[]  KtOutMin=[]  KtOutMax=[]  IntegratorOutMin=[]  IntegratorOutMax=[]  FilterOutMin=[]  FilterOutMax=[]  SumI1OutMin=[]  SumI1OutMax=[]  SumI2OutMin=[]  SumI2OutMax=[]  SumI3OutMin=[]  SumI3OutMax=[]  SumI4OutMin=[]  SumI4OutMax=[]  SumDOutMin=[]  SumDOutMax=[]  DifferentiatorOutMin=[]  DifferentiatorOutMax=[]  FilterDiffOutCoefMin=[]  FilterDiffOutCoefMax=[]  ReciprocalOutMin=[]  ReciprocalOutMax=[]  SumDenOutMin=[]  SumDenOutMax=[]  SumNumOutMin=[]  SumNumOutMax=[]  DivideOutMin=[]  DivideOutMax=[]  UdiffTsProdOutMin=[]  UdiffTsProdOutMax=[]  NTsProdOutMin=[]  NTsProdOutMax=[]  UintegralTsProdOutMin=[]  UintegralTsProdOutMax=[]  UngainTsProdOutMin=[]  UngainTsProdOutMax=[]  IntegratorContinuousStateAttributes=''  IntegratorStateMustResolveToSignalObject=off  IntegratorRTWStateStorageClass=Auto  FilterContinuousStateAttributes=''  FilterStateMustResolveToSignalObject=off  FilterRTWStateStorageClass=Auto  ParallelPVariant=ExternalParameters  IdealPVariant=Disabled  IVariant=ExternalParameters  DVariant=ExternalParameters  IntegratorVariant=Continuous  SatVariant=Disabled  AWVariant=Passthrough  PCopyVariant=Disabled  TRVariant=Disabled  FdbkBlocksVariant=Forward  IdealPFdbkVariant=Disabled  SatFdbkVariant=Disabled  DerivativeFilterVariant=ContFilter  NVariant=ExternalParameters  NCopyVariant=Disabled  FilterICVariant=InternalICsFilter  IntegratorICVariant=InternalICs  ExternalResetVariant=Disabled  TRSumVariant=Passthrough  SumFdbkVariant=Disabled  SumVariant=Sum_PID  TsampFilterVariant=InternalTs  TsampNgainVariant=Passthrough  TsampIntegralVariant=Passthrough  ExternalSaturationOutDataTypeStr=Inherit: Same as second input
  pitch PID : pid_lib/PID Controller  Controller=PID  Form=Parallel  TimeDomain=Continuous-time  UseExternalTs=off  SampleTime=-1  IntegratorMethod=Forward Euler  FilterMethod=Forward Euler  ControllerParametersSource=external  P=0.01  I=0  D=1  UseFilter=on  N=100  TunerSelectOption=Transfer Function Based (PID Tuner App)  InitialConditionSource=internal  InitialConditionForIntegrator=0  InitialConditionForFilter=0  DifferentiatorICPrevScaledInput=0  ExternalReset=none  TrackingMode=off  Kt=1  LimitOutput=off  SatLimitsSource=internal  UpperSaturationLimit=inf  LowerSaturationLimit=-inf  LinearizeAsGain=on  AntiWindupMode=none  Kb=1  POutMin=[]  POutMax=[]  IOutMin=[]  IOutMax=[]  DOutMin=[]  DOutMax=[]  NOutMin=[]  NOutMax=[]  SumOutMin=[]  SumOutMax=[]  SaturationOutMin=[]  SaturationOutMax=[]  PParamMin=[]  PParamMax=[]  IParamMin=[]  IParamMax=[]  DParamMin=[]  DParamMax=[]  NParamMin=[]  NParamMax=[]  KbParamMin=[]  KbParamMax=[]  KtParamMin=[]  KtParamMax=[]  KbOutMin=[]  KbOutMax=[]  KtOutMin=[]  KtOutMax=[]  IntegratorOutMin=[]  IntegratorOutMax=[]  FilterOutMin=[]  FilterOutMax=[]  SumI1OutMin=[]  SumI1OutMax=[]  SumI2OutMin=[]  SumI2OutMax=[]  SumI3OutMin=[]  SumI3OutMax=[]  SumI4OutMin=[]  SumI4OutMax=[]  SumDOutMin=[]  SumDOutMax=[]  DifferentiatorOutMin=[]  DifferentiatorOutMax=[]  FilterDiffOutCoefMin=[]  FilterDiffOutCoefMax=[]  ReciprocalOutMin=[]  ReciprocalOutMax=[]  SumDenOutMin=[]  SumDenOutMax=[]  SumNumOutMin=[]  SumNumOutMax=[]  DivideOutMin=[]  DivideOutMax=[]  UdiffTsProdOutMin=[]  UdiffTsProdOutMax=[]  NTsProdOutMin=[]  NTsProdOutMax=[]  UintegralTsProdOutMin=[]  UintegralTsProdOutMax=[]  UngainTsProdOutMin=[]  UngainTsProdOutMax=[]  IntegratorContinuousStateAttributes=''  IntegratorStateMustResolveToSignalObject=off  IntegratorRTWStateStorageClass=Auto  FilterContinuousStateAttributes=''  FilterStateMustResolveToSignalObject=off  FilterRTWStateStorageClass=Auto  ParallelPVariant=ExternalParameters  IdealPVariant=Disabled  IVariant=ExternalParameters  DVariant=ExternalParameters  IntegratorVariant=Continuous  SatVariant=Disabled  AWVariant=Passthrough  PCopyVariant=Disabled  TRVariant=Disabled  FdbkBlocksVariant=Forward  IdealPFdbkVariant=Disabled  SatFdbkVariant=Disabled  DerivativeFilterVariant=ContFilter  NVariant=ExternalParameters  NCopyVariant=Disabled  FilterICVariant=InternalICsFilter  IntegratorICVariant=InternalICs  ExternalResetVariant=Disabled  TRSumVariant=Passthrough  SumFdbkVariant=Disabled  SumVariant=Sum_PID  TsampFilterVariant=InternalTs  TsampNgainVariant=Passthrough  TsampIntegralVariant=Passthrough  ExternalSaturationOutDataTypeStr=Inherit: Same as second input
  yaw PID : pid_lib/PID Controller  Controller=PID  Form=Parallel  TimeDomain=Continuous-time  UseExternalTs=off  SampleTime=-1  IntegratorMethod=Forward Euler  FilterMethod=Forward Euler  ControllerParametersSource=external  P=0.01  I=0  D=1  UseFilter=on  N=100  TunerSelectOption=Transfer Function Based (PID Tuner App)  InitialConditionSource=internal  InitialConditionForIntegrator=0  InitialConditionForFilter=0  DifferentiatorICPrevScaledInput=0  ExternalReset=none  TrackingMode=off  Kt=1  LimitOutput=off  SatLimitsSource=internal  UpperSaturationLimit=inf  LowerSaturationLimit=-inf  LinearizeAsGain=on  AntiWindupMode=none  Kb=1  POutMin=[]  POutMax=[]  IOutMin=[]  IOutMax=[]  DOutMin=[]  DOutMax=[]  NOutMin=[]  NOutMax=[]  SumOutMin=[]  SumOutMax=[]  SaturationOutMin=[]  SaturationOutMax=[]  PParamMin=[]  PParamMax=[]  IParamMin=[]  IParamMax=[]  DParamMin=[]  DParamMax=[]  NParamMin=[]  NParamMax=[]  KbParamMin=[]  KbParamMax=[]  KtParamMin=[]  KtParamMax=[]  KbOutMin=[]  KbOutMax=[]  KtOutMin=[]  KtOutMax=[]  IntegratorOutMin=[]  IntegratorOutMax=[]  FilterOutMin=[]  FilterOutMax=[]  SumI1OutMin=[]  SumI1OutMax=[]  SumI2OutMin=[]  SumI2OutMax=[]  SumI3OutMin=[]  SumI3OutMax=[]  SumI4OutMin=[]  SumI4OutMax=[]  SumDOutMin=[]  SumDOutMax=[]  DifferentiatorOutMin=[]  DifferentiatorOutMax=[]  FilterDiffOutCoefMin=[]  FilterDiffOutCoefMax=[]  ReciprocalOutMin=[]  ReciprocalOutMax=[]  SumDenOutMin=[]  SumDenOutMax=[]  SumNumOutMin=[]  SumNumOutMax=[]  DivideOutMin=[]  DivideOutMax=[]  UdiffTsProdOutMin=[]  UdiffTsProdOutMax=[]  NTsProdOutMin=[]  NTsProdOutMax=[]  UintegralTsProdOutMin=[]  UintegralTsProdOutMax=[]  UngainTsProdOutMin=[]  UngainTsProdOutMax=[]  IntegratorContinuousStateAttributes=''  IntegratorStateMustResolveToSignalObject=off  IntegratorRTWStateStorageClass=Auto  FilterContinuousStateAttributes=''  FilterStateMustResolveToSignalObject=off  FilterRTWStateStorageClass=Auto  ParallelPVariant=ExternalParameters  IdealPVariant=Disabled  IVariant=ExternalParameters  DVariant=ExternalParameters  IntegratorVariant=Continuous  SatVariant=Disabled  AWVariant=Passthrough  PCopyVariant=Disabled  TRVariant=Disabled  FdbkBlocksVariant=Forward  IdealPFdbkVariant=Disabled  SatFdbkVariant=Disabled  DerivativeFilterVariant=ContFilter  NVariant=ExternalParameters  NCopyVariant=Disabled  FilterICVariant=InternalICsFilter  IntegratorICVariant=InternalICs  ExternalResetVariant=Disabled  TRSumVariant=Passthrough  SumFdbkVariant=Disabled  SumVariant=Sum_PID  TsampFilterVariant=InternalTs  TsampNgainVariant=Passthrough  TsampIntegralVariant=Passthrough  ExternalSaturationOutDataTypeStr=Inherit: Same as second input
  x pid : Outport  Unit=1
  pitch pid : Outport  Port=2  Unit=1
  yaw pid : Outport  Port=3  Unit=1
  wires:
  P/1 -> Gain4/1, pitch PID/2, forward PID/2
  N/1 -> yaw PID/5, pitch PID/5, forward PID/5
  I/1 -> pitch PID/3, yaw PID/3, forward PID/3
  D/1 -> pitch PID/4, yaw PID/4, forward PID/4
  pitch error/1 -> pitch PID/1
  forward PID/1 -> x pid/1
  yaw error/1 -> yaw PID/1
  forward speed error/1 -> forward PID/1
  Gain4/1 -> yaw PID/2
  pitch PID/1 -> pitch pid/1
  yaw PID/1 -> yaw pid/1

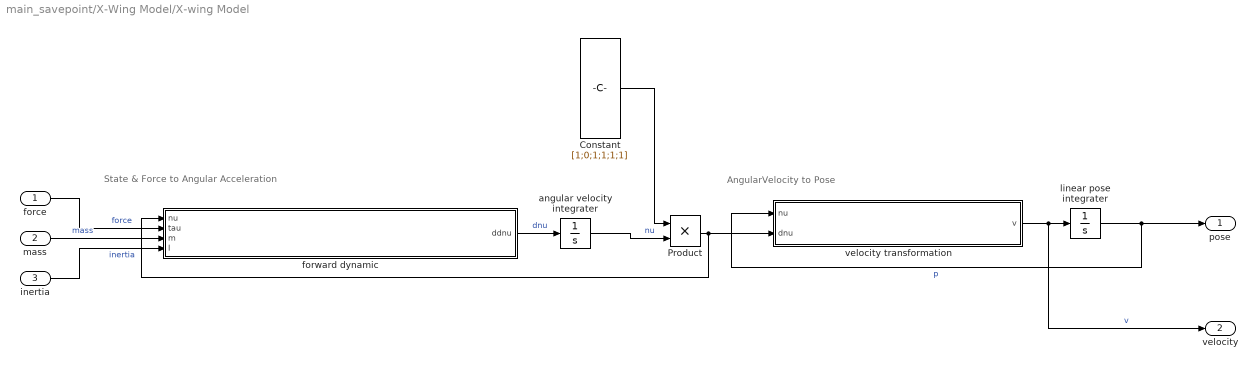
== system main_savepoint/X-Wing Model/X-wing Model ==
  note: State & Force to Angular Acceleration
  note: AngularVelocity to Pose
  force : Inport
  mass : Inport  Port=2
  inertia : Inport  Port=3
  Constant : Constant  Value=[1;0;1;1;1;1]  VectorParams1D=off
  Product : Product
  angular velocity integrater : Integrator  InitialCondition=[0;0;0;0;0;0]
  forward dynamic : MATLAB Function  TreatAsAtomicUnit=on
  linear pose integrater : Integrator  InitialCondition=[0;0;1.705;0.0;0.0;0.0]
  velocity transformation : MATLAB Function  TreatAsAtomicUnit=on
  pose : Outport  PortDimensions=6
  velocity : Outport  Port=2  PortDimensions=6
  wires:
  velocity transformation/1(v) -> velocity/1, linear pose integrater/1  "v"
  forward dynamic/1(ddnu) -> angular velocity integrater/1  "dnu"
  linear pose integrater/1 -> pose/1, velocity transformation/1(nu)  "p"
  angular velocity integrater/1 -> Product/2  "nu"
  mass/1 -> forward dynamic/3(m)  "mass"
  inertia/1 -> forward dynamic/4(I)  "inertia"
  force/1 -> forward dynamic/2(tau)  "force"
  Product/1 -> velocity transformation/2(dnu), forward dynamic/1(nu)
  Constant/1 -> Product/1

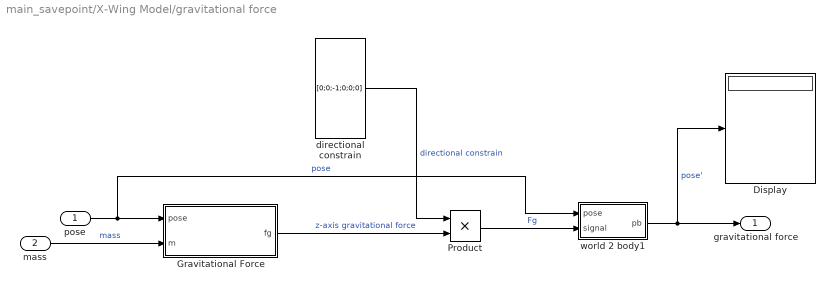
== system main_savepoint/X-Wing Model/gravitational force ==
  pose : Inport
  mass : Inport  Port=2
  Display : Display
  Gravitational Force : MATLAB Function  TreatAsAtomicUnit=on
  Product : Product
  directional constrain : Constant  Value=[0;0;-1;0;0;0]  VectorParams1D=off
  world 2 body1 : MATLAB Function  TreatAsAtomicUnit=on
  gravitational force : Outport  PortDimensions=6
  wires:
  mass/1 -> Gravitational Force/2(m)  "mass"
  directional constrain/1 -> Product/1  "directional constrain"
  Gravitational Force/1(fg) -> Product/2  "z-axis gravitational force"
  pose/1 -> world 2 body1/1(pose), Gravitational Force/1(pose)  "pose"
  Product/1 -> world 2 body1/2(signal)  "Fg"
  world 2 body1/1(pb) -> Display/1, gravitational force/1  "pose'"

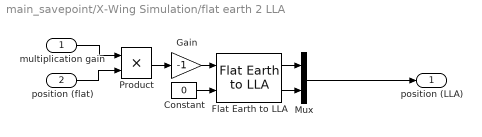
== system main_savepoint/X-Wing Simulation/flat earth 2 LLA ==
  multiplication gain : Inport
  position (flat) : Inport  Port=2
  Constant : Constant  Value=0
  Flat Earth to LLA : aerolibtransform2/Flat Earth to LLA  units=Metric (MKS)  ptype=Earth (WGS84)  F=1/298.257223563  R=6378137  refPosPort=off  LL0=[-45 83.1]  psi=90
  Gain : Gain  Gain=-1
  Mux : Mux  Inputs=2
  Product : Product
  position (LLA) : Outport
  wires:
  Product/1 -> Gain/1
  Constant/1 -> Flat Earth to LLA/2
  Flat Earth to LLA/1 -> Mux/1
  Flat Earth to LLA/2 -> Mux/2
  position (flat)/1 -> Product/2
  Gain/1 -> Flat Earth to LLA/1
  Mux/1 -> position (LLA)/1
  multiplication gain/1 -> Product/1

== matlab function main_savepoint/X-Wing Model/gravitational force/Gravitational Force ==
  data: pose input; fg output; m input
function fg = gravitational_force(pose,m)


G = 6.67259*10^-11; % gravitational constant < Nm2/kg2 >
M = 5.98*10^24; % earth mass <kg>
R = 6.38*10^6; % average earth radius <m>
r = R + pose(3); % distance from the surface <m>

fg = G*m*M/(r*r); % F = Gmm/r^2

end

== matlab function main_savepoint/X-Wing Model/X-wing Model/forward dynamic ==
  data: nu input; ddnu output; tau input; m input; I input
function ddnu = forwardDynamic(nu,tau,m,I)

% extracted state variable
omega = nu(4:6); % droll dpitch dyaw

% force 
F = [0;0;0;0;0;0]+tau;

% constant
M = [m*eye(3) zeros(3,3);zeros(3,3) I]; % mass/inertia matrix
C = [m*skewy(omega) zeros(3,3);zeros(3,3) -skewy(I*omega)];

ddnu = inv(M)*(F-C*nu);
end

function s = skewy(x)
    s = zeros(3,3);
    s(1,2) = -x(3);
    s(1,3) = x(2);
    s(2,1) = x(3);
    s(2,3) = -x(1);
    s(3,1) = -x(2);
    s(3,2) = x(1);
end

== matlab function main_savepoint/state preprocessing/world 2 body2 ==
  data: pb output; pose input; signal input
function pb= fcn(pose,signal)
R = rotz(rad2deg(pose(6)))*roty(rad2deg(pose(5)))*rotx(rad2deg(pose(4)));
pb = [R.'*signal(1:3);signal(4:6)];

== matlab function main_savepoint/X-Wing Model/X-wing Model/velocity transformation ==
  data: nu input; dnu input; v output
function v = velocityTrans(nu,dnu)
    roll = nu(4);
    pitch = nu(5);
    yaw = nu(6);
    Rx = [1 0 0;0 cos(roll) -sin(roll); 0 sin(roll) cos(roll)];
    Ry = [cos(pitch) 0 sin(pitch); 0 1 0; -sin(pitch) 0 cos(pitch)];
    Rz = [cos(yaw) -sin(yaw) 0; sin(yaw) cos(yaw) 0;0 0 1];
    R = Rz*Ry*Rx;
    T = [1 sin(roll)*tan(pitch) cos(roll)*tan(pitch); 0 cos(roll) -sin(roll); 0 sin(roll)/cos(pitch) cos(roll)/cos(pitch)];
    J = [R zeros(3,3);zeros(3,3) T];
    v = J*dnu;
end

== matlab function main_savepoint/X-Wing Simulation/MATLAB Function ==
  data: pose input; pose_ output
function pose_ = simulation_interface(pose)
R = 6.38*10^6; % average earth radius <m>
gain = 1e3;
x = pose(1); % flip the x-axis;
y = pose(2);
z = pose(3);
position = [x;y;z];%+[-45;83.1;0];
pose_ = [position;-pose(5);-pose(4);(-1.57-pose(6))];
end

== matlab function main_savepoint/X-Wing Model/gravitational force/world 2 body1 ==
  data: pb output; pose input; signal input
function pb= fcn(pose,signal)
R = rotz(rad2deg(pose(6)))*roty(rad2deg(pose(5)))*rotx(rad2deg(pose(4)));
pb = [R.'*(signal(1:3));signal(4:6)];

== matlab function main_savepoint/state preprocessing/world 2 body1 ==
  data: pb output; pose input; signal input
function pb= fcn(pose,signal)
R = rotz(rad2deg(pose(6)))*roty(rad2deg(pose(5)))*rotx(rad2deg(pose(4)));
pb = [R.'*signal(1:3);signal(4:6)];
